simulink model "rlMultiAgentPFC"  (R2022a)
settings: Solver=VariableStepAuto  StartTime=0.0  StopTime=Tf  FixedStep=1e-3  RelTol=1e-3
values from neighbouring files (symbols this model uses):
  Ts = 100    [MultiAgent_initiateSAC.m]    (also in control_velocity.m; initiate.m; initiateHybrid.m = 50; initiateSAC.m)
undefined symbols (not defined in the file or in its folder): amax_ego, amin_ego, Cf, Cr, D_default, DiscIntNeverNeededParam, e1_initial, e2_initial, Iz, lf, lr, m, rho, t_gap, tau, umax_ego, umin_ego, v0_ego, v0_lead, v_set, x0_ego, x0_lead
libraries: simulink x5, rllib x2
settings Model: Creator=The MathWorks, Inc.  LastModifiedBy=The MathWorks, Inc.
settings SolverCC: AlgebraicLoopSolver=TrustRegion
settings DataIOCC: SaveOutput=off  SignalLogging=off  DSMLogging=off  SaveTime=off  ReturnWorkspaceOutputs=off
settings DebuggingCC: ParameterPrecisionLossMsg=none  UnconnectedInputMsg=warning  UnconnectedOutputMsg=warning  UnconnectedLineMsg=warning  SFMachineParentedDataDiag=warning  ArithmeticOperatorsInVariantConditions=warning
settings SFSimCC: SimUseLocalCustomCode=off
settings RTWCC: RTWUseLocalCustomCode=off  DLArmComputeVersion=19.05

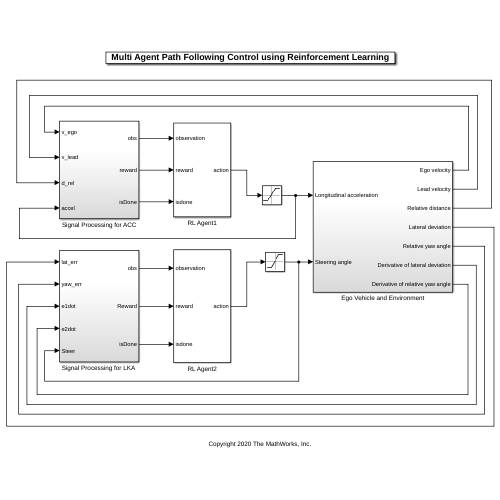
[thumbnail: Simulink's stored preview of the top-level diagram]
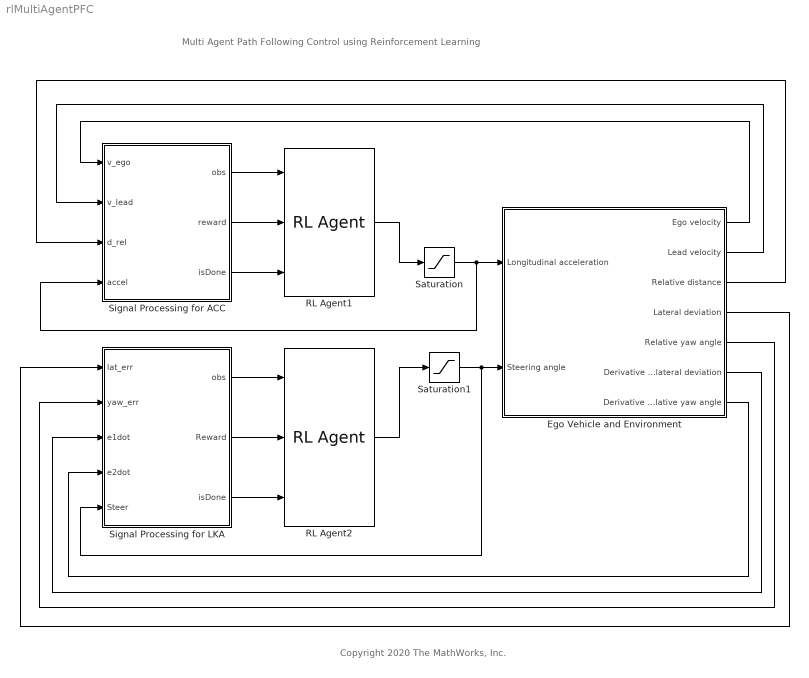
== system rlMultiAgentPFC ==
  note: Copyright 2020 The MathWorks, Inc.
  note: Multi Agent Path Following Control using Reinforcement Learning
  Ego Vehicle and Environment : Subsystem
  RL Agent1 : rllib/RL Agent  Agent=agent1  ExternalActionAsInput=off  ProvideLastAction=off  ProvideCumRwd=off  TreatAsDirectFeedthrough=on  UseStrictObservationDataTypes=off
  RL Agent2 : rllib/RL Agent  Agent=agent2  ExternalActionAsInput=off  ProvideLastAction=off  ProvideCumRwd=off  TreatAsDirectFeedthrough=on  UseStrictObservationDataTypes=off
  Saturation : Saturate  UpperLimit=amax_ego  LowerLimit=amin_ego
  Saturation1 : Saturate  UpperLimit=umax_ego  LowerLimit=umin_ego
  Signal Processing for ACC : Subsystem
  "Signal Processing for LKA " : Subsystem
  wires:
  Saturation/1 -> Signal Processing for ACC/4(accel), Ego Vehicle and Environment/1(Longitudinal acceleration)
  Saturation1/1 -> "Signal Processing for LKA "/5(Steer), Ego Vehicle and Environment/2(Steering angle)
  RL Agent1/1 -> Saturation/1
  RL Agent2/1 -> Saturation1/1
  Signal Processing for ACC/1(obs) -> RL Agent1/1
  Signal Processing for ACC/2(reward) -> RL Agent1/2
  Signal Processing for ACC/3(isDone) -> RL Agent1/3
  "Signal Processing for LKA "/1(obs) -> RL Agent2/1
  "Signal Processing for LKA "/2(Reward) -> RL Agent2/2
  "Signal Processing for LKA "/3(isDone) -> RL Agent2/3
  Ego Vehicle and Environment/3(Relative distance) -> Signal Processing for ACC/3(d_rel)
  Ego Vehicle and Environment/2(Lead velocity) -> Signal Processing for ACC/2(v_lead)
  Ego Vehicle and Environment/1(Ego velocity) -> Signal Processing for ACC/1(v_ego)
  Ego Vehicle and Environment/7(Derivative of relative yaw angle) -> "Signal Processing for LKA "/4(e2dot)
  Ego Vehicle and Environment/6(Derivative of lateral deviation) -> "Signal Processing for LKA "/3("e1dot ")
  Ego Vehicle and Environment/5(Relative yaw angle) -> "Signal Processing for LKA "/2(yaw_err)
  Ego Vehicle and Environment/4(Lateral deviation) -> "Signal Processing for LKA "/1(lat_err)

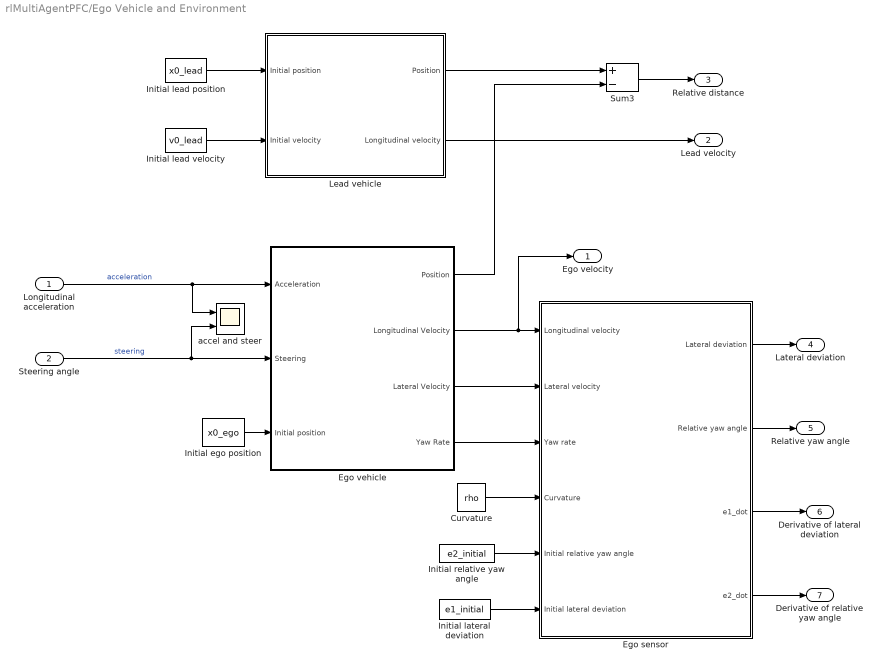
== system rlMultiAgentPFC/Ego Vehicle and Environment ==
  Longitudinal acceleration : Inport
  Steering angle : Inport  Port=2
  Curvature : Constant  Value=rho
  Ego sensor : Subsystem
  Ego vehicle : Subsystem
  Initial ego position : Constant  Value=x0_ego
  Initial lateral deviation : Constant  Value=e1_initial
  Initial lead position : Constant  Value=x0_lead
  Initial lead velocity : Constant  Value=v0_lead
  Initial relative yaw angle : Constant  Value=e2_initial
  Lead vehicle : Subsystem
  Sum3 : Sum  Inputs=+-
  accel and steer : Scope  NumInputPorts=2
  Ego velocity : Outport  VectorParamsAs1DForOutWhenUnconnected=off
  Lead velocity : Outport  Port=2  VectorParamsAs1DForOutWhenUnconnected=off
  Relative distance : Outport  Port=3  VectorParamsAs1DForOutWhenUnconnected=off
  Lateral deviation : Outport  Port=4  VectorParamsAs1DForOutWhenUnconnected=off
  Relative yaw angle : Outport  Port=5  VectorParamsAs1DForOutWhenUnconnected=off
  Derivative of lateral deviation : Outport  Port=6  VectorParamsAs1DForOutWhenUnconnected=off
  Derivative of relative yaw angle : Outport  Port=7  VectorParamsAs1DForOutWhenUnconnected=off
  wires:
  Ego vehicle/3(Lateral Velocity) -> Ego sensor/2(Lateral velocity)
  Ego vehicle/4(Yaw Rate) -> Ego sensor/3(Yaw rate)
  Longitudinal acceleration/1 -> accel and steer/1, Ego vehicle/1(Acceleration)  "acceleration"
  Ego sensor/1(Lateral deviation) -> Lateral deviation/1
  Ego vehicle/2(Longitudinal Velocity) -> Ego velocity/1, Ego sensor/1(Longitudinal velocity)
  Steering angle/1 -> accel and steer/2, Ego vehicle/2(Steering)  "steering"
  Ego sensor/2(Relative yaw angle) -> Relative yaw angle/1
  Initial lateral deviation/1 -> Ego sensor/6(Initial lateral deviation)
  Initial ego position/1 -> Ego vehicle/3(Initial position)
  Curvature/1 -> Ego sensor/4(Curvature)
  Initial relative yaw angle/1 -> Ego sensor/5(Initial relative yaw angle)
  Initial lead velocity/1 -> Lead vehicle/2(Initial velocity)
  Initial lead position/1 -> Lead vehicle/1(Initial position)
  Lead vehicle/1(Position) -> Sum3/1
  Ego vehicle/1(Position) -> Sum3/2
  Sum3/1 -> Relative distance/1
  Lead vehicle/2(Longitudinal velocity) -> Lead velocity/1
  Ego sensor/3(e1_dot) -> Derivative of lateral deviation/1
  Ego sensor/4(e2_dot) -> Derivative of relative yaw angle/1

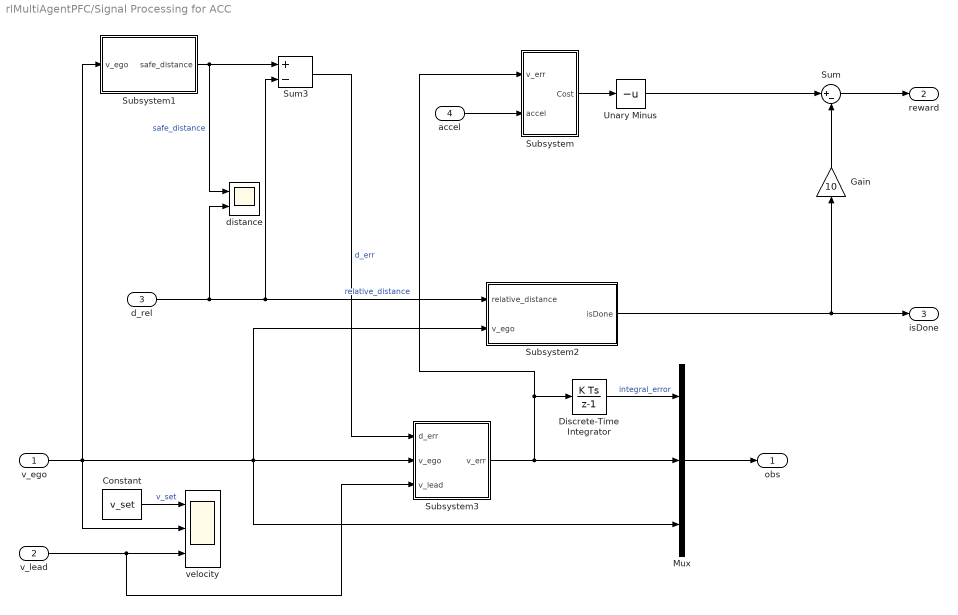
== system rlMultiAgentPFC/Signal Processing for ACC ==
  v_ego : Inport
  v_lead : Inport  Port=2
  d_rel : Inport  Port=3
  accel : Inport  Port=4
  Constant : Constant  Value=v_set
  Discrete-Time Integrator : DiscreteIntegrator  SampleTime=-1  ICPrevOutput=DiscIntNeverNeededParam  ICPrevScaledInput=DiscIntNeverNeededParam
  Gain : Gain  Gain=10
  Mux : Mux  Inputs=3
  Subsystem : Subsystem
  Subsystem1 : Subsystem
  Subsystem2 : Subsystem
  Subsystem3 : Subsystem
  Sum : Sum  Inputs=|+-
  Sum3 : Sum  Inputs=+-
  Unary Minus : UnaryMinus
  distance : Scope  NumInputPorts=2
  velocity : Scope  NumInputPorts=3
  obs : Outport  VectorParamsAs1DForOutWhenUnconnected=off
  reward : Outport  Port=2  VectorParamsAs1DForOutWhenUnconnected=off
  isDone : Outport  Port=3  VectorParamsAs1DForOutWhenUnconnected=off
  wires:
  Constant/1 -> velocity/1  "v_set"
  v_lead/1 -> velocity/3, Subsystem3/3(v_lead)
  Discrete-Time Integrator/1 -> Mux/1  "integral_error"
  Mux/1 -> obs/1
  v_ego/1 -> velocity/2, Subsystem3/2(v_ego), Mux/3, Subsystem2/2(v_ego), Subsystem1/1(v_ego)
  d_rel/1 -> distance/2, Sum3/2, Subsystem2/1(relative_distance)  "relative_distance"
  Subsystem/1(Cost) -> Unary Minus/1
  Sum3/1 -> Subsystem3/1(d_err)  "d_err"
  Subsystem1/1(safe_distance) -> distance/1, Sum3/1  "safe_distance"
  accel/1 -> Subsystem/2(accel)
  Subsystem3/1(v_err) -> Subsystem/1(v_err), Discrete-Time Integrator/1, Mux/2
  Subsystem2/1(isDone) -> isDone/1, Gain/1
  Unary Minus/1 -> Sum/1
  Gain/1 -> Sum/2
  Sum/1 -> reward/1

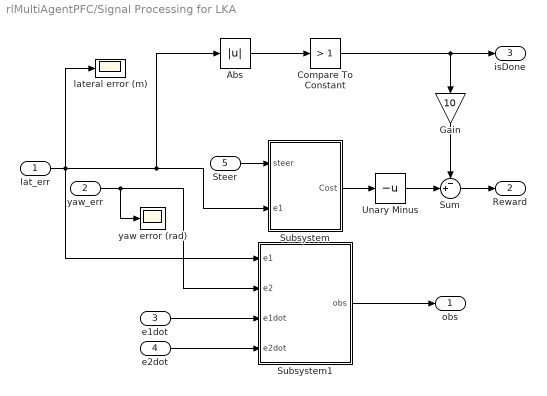
== system rlMultiAgentPFC/Signal Processing for LKA  ==
  lat_err : Inport
  yaw_err : Inport  Port=2
  "e1dot " : Inport  Port=3
  e2dot : Inport  Port=4
  Steer : Inport  Port=5
  Abs : Abs  SaturateOnIntegerOverflow=off
  Compare To Constant : simulink/Logic and Bit Operations/Compare To Constant  relop=>  const=1  OutDataTypeStr=boolean
  Gain : Gain  Gain=10
  Subsystem : Subsystem
  Subsystem1 : Subsystem
  Sum : Sum  Inputs=-+|
  Unary Minus : UnaryMinus
  lateral error (m) : Scope
  yaw error (rad) : Scope
  obs : Outport  VectorParamsAs1DForOutWhenUnconnected=off
  Reward : Outport  Port=2  VectorParamsAs1DForOutWhenUnconnected=off
  isDone : Outport  Port=3  VectorParamsAs1DForOutWhenUnconnected=off
  wires:
  Subsystem/1(Cost) -> Unary Minus/1
  lat_err/1 -> Subsystem1/1(e1), Subsystem/2(e1), Abs/1, lateral error (m)/1
  yaw_err/1 -> yaw error (rad)/1, Subsystem1/2(e2)
  Abs/1 -> Compare To Constant/1
  Subsystem1/1(obs) -> obs/1
  "e1dot "/1 -> Subsystem1/3(e1dot)
  e2dot/1 -> Subsystem1/4(e2dot)
  Steer/1 -> Subsystem/1(steer)
  Compare To Constant/1 -> Gain/1, isDone/1
  Gain/1 -> Sum/1
  Sum/1 -> Reward/1
  Unary Minus/1 -> Sum/2

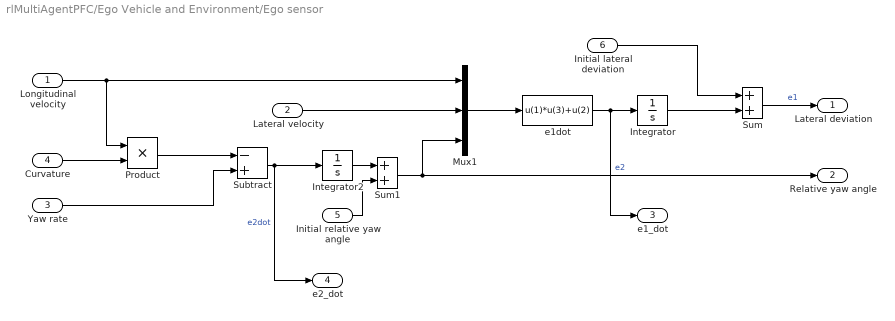
== system rlMultiAgentPFC/Ego Vehicle and Environment/Ego sensor ==
  Longitudinal velocity : Inport
  Lateral velocity : Inport  Port=2
  Yaw rate : Inport  Port=3
  Curvature : Inport  Port=4
  Initial relative yaw angle : Inport  Port=5
  Initial lateral deviation : Inport  Port=6
  Integrator : Integrator
  Integrator2 : Integrator
  Mux1 : Mux  Inputs=[1 1 1]
  Product : Product
  Subtract : Sum  Inputs=-+
  Sum : Sum
  Sum1 : Sum
  e1dot : Fcn  Expr=u(1)*u(3)+u(2)
  Lateral deviation : Outport  VectorParamsAs1DForOutWhenUnconnected=off
  Relative yaw angle : Outport  Port=2  VectorParamsAs1DForOutWhenUnconnected=off
  e1_dot : Outport  Port=3  VectorParamsAs1DForOutWhenUnconnected=off
  e2_dot : Outport  Port=4  VectorParamsAs1DForOutWhenUnconnected=off
  wires:
  Curvature/1 -> Product/2
  Sum1/1 -> Mux1/3, Relative yaw angle/1  "e2"
  Mux1/1 -> e1dot/1
  Initial lateral deviation/1 -> Sum/1
  e1dot/1 -> e1_dot/1, Integrator/1
  Integrator/1 -> Sum/2
  Longitudinal velocity/1 -> Product/1, Mux1/1
  Lateral velocity/1 -> Mux1/2
  Sum/1 -> Lateral deviation/1  "e1"
  Integrator2/1 -> Sum1/1
  Initial relative yaw angle/1 -> Sum1/2
  Product/1 -> Subtract/1
  Yaw rate/1 -> Subtract/2
  Subtract/1 -> e2_dot/1, Integrator2/1  "e2dot"

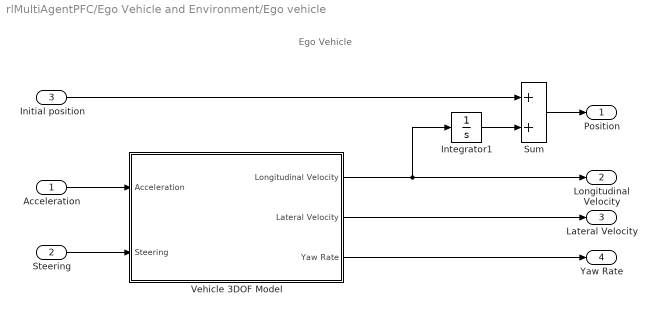
== system rlMultiAgentPFC/Ego Vehicle and Environment/Ego vehicle ==
  note: Ego Vehicle
  Acceleration : Inport
  Steering : Inport  Port=2
  Initial position : Inport  Port=3
  Integrator1 : Integrator
  Sum : Sum
  Vehicle 3DOF Model : Subsystem
  Position : Outport  VectorParamsAs1DForOutWhenUnconnected=off
  Longitudinal Velocity : Outport  Port=2  VectorParamsAs1DForOutWhenUnconnected=off
  Lateral Velocity : Outport  Port=3  VectorParamsAs1DForOutWhenUnconnected=off
  Yaw Rate : Outport  Port=4  VectorParamsAs1DForOutWhenUnconnected=off
  wires:
  Integrator1/1 -> Sum/2
  Initial position/1 -> Sum/1
  Sum/1 -> Position/1
  Acceleration/1 -> Vehicle 3DOF Model/1(Acceleration)
  Steering/1 -> Vehicle 3DOF Model/2(Steering)
  Vehicle 3DOF Model/2(Lateral Velocity) -> Lateral Velocity/1
  Vehicle 3DOF Model/3(Yaw Rate) -> Yaw Rate/1
  Vehicle 3DOF Model/1(Longitudinal Velocity) -> Longitudinal Velocity/1, Integrator1/1

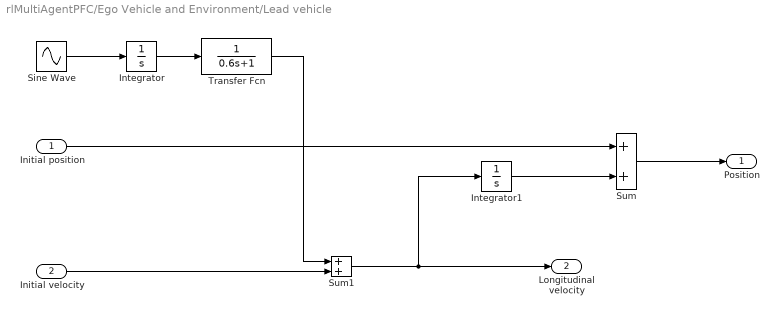
== system rlMultiAgentPFC/Ego Vehicle and Environment/Lead vehicle ==
  Initial position : Inport
  Initial velocity : Inport  Port=2
  Integrator : Integrator
  Integrator1 : Integrator
  Sine Wave : Sin  Amplitude=0.6  Frequency=0.2  SampleTime=Ts
  Sum : Sum
  Sum1 : Sum
  Transfer Fcn : TransferFcn  Denominator=[0.6 1]
  Position : Outport  VectorParamsAs1DForOutWhenUnconnected=off
  Longitudinal velocity : Outport  Port=2  VectorParamsAs1DForOutWhenUnconnected=off
  wires:
  Transfer Fcn/1 -> Sum1/1
  Initial velocity/1 -> Sum1/2
  Sum/1 -> Position/1
  Integrator/1 -> Transfer Fcn/1
  Sum1/1 -> Integrator1/1, Longitudinal velocity/1
  Sine Wave/1 -> Integrator/1
  Initial position/1 -> Sum/1
  Integrator1/1 -> Sum/2

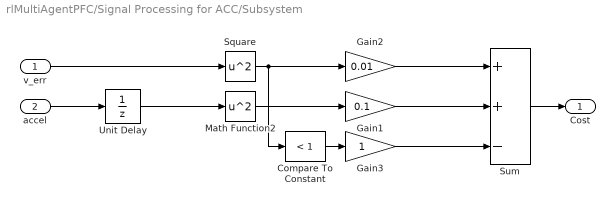
== system rlMultiAgentPFC/Signal Processing for ACC/Subsystem ==
  v_err : Inport
  accel : Inport  Port=2
  Compare To Constant : simulink/Logic and Bit Operations/Compare To Constant  relop=<  const=1  OutDataTypeStr=boolean
  Gain1 : Gain  Gain=0.1
  Gain2 : Gain  Gain=0.01
  Gain3 : Gain
  Math Function2 : Math  Operator=square  SignedPower=on
  Square : Math  Operator=square  SignedPower=on
  Sum : Sum  Inputs=++-
  Unit Delay : UnitDelay  SampleTime=-1  HasFrameUpgradeWarning=on
  Cost : Outport  VectorParamsAs1DForOutWhenUnconnected=off
  wires:
  v_err/1 -> Square/1
  Math Function2/1 -> Gain1/1
  accel/1 -> Unit Delay/1
  Sum/1 -> Cost/1
  Square/1 -> Compare To Constant/1, Gain2/1
  Unit Delay/1 -> Math Function2/1
  Gain2/1 -> Sum/1
  Gain1/1 -> Sum/2
  Compare To Constant/1 -> Gain3/1
  Gain3/1 -> Sum/3

== system rlMultiAgentPFC/Signal Processing for ACC/Subsystem1 ==
  v_ego : Inport
  Default Spacing : Constant  Value=D_default  SampleTime=Ts
  Product : Product
  Sum2 : Sum
  Time Gap : Constant  Value=t_gap  SampleTime=Ts
  safe_distance : Outport  VectorParamsAs1DForOutWhenUnconnected=off
  wires:
  Sum2/1 -> safe_distance/1
  Product/1 -> Sum2/2
  Time Gap/1 -> Product/2
  Default Spacing/1 -> Sum2/1
  v_ego/1 -> Product/1

== system rlMultiAgentPFC/Signal Processing for ACC/Subsystem2 ==
  relative_distance : Inport
  v_ego : Inport  Port=2
  Logical Operator : Logic  Operator=OR  AllPortsSameDT=off  OutDataTypeStr=boolean
  Relative Distance : simulink/Logic and Bit Operations/Compare To Constant  relop=<  const=0  OutDataTypeStr=boolean
  Velocity : simulink/Logic and Bit Operations/Compare To Constant  relop=<  const=0.5  OutDataTypeStr=boolean
  isDone : Outport  VectorParamsAs1DForOutWhenUnconnected=off
  wires:
  Velocity/1 -> Logical Operator/2
  Relative Distance/1 -> Logical Operator/1
  relative_distance/1 -> Relative Distance/1
  Logical Operator/1 -> isDone/1
  v_ego/1 -> Velocity/1

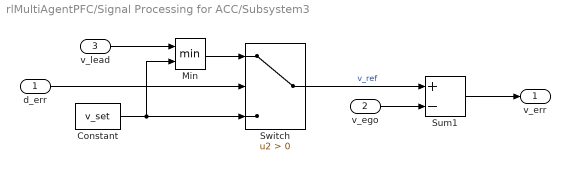
== system rlMultiAgentPFC/Signal Processing for ACC/Subsystem3 ==
  d_err : Inport
  v_ego : Inport  Port=2
  v_lead : Inport  Port=3
  Constant : Constant  Value=v_set
  Min : MinMax  Inputs=2
  Sum1 : Sum  Inputs=+-
  Switch : Switch  Criteria=u2 > Threshold  SaturateOnIntegerOverflow=off  InputSameDT=off
  v_err : Outport  VectorParamsAs1DForOutWhenUnconnected=off
  wires:
  Sum1/1 -> v_err/1
  v_ego/1 -> Sum1/2
  Switch/1 -> Sum1/1  "v_ref"
  d_err/1 -> Switch/2
  Constant/1 -> Min/2, Switch/3
  Min/1 -> Switch/1
  v_lead/1 -> Min/1

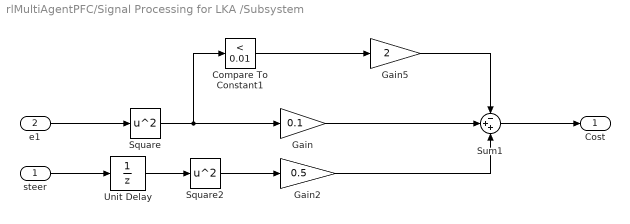
== system rlMultiAgentPFC/Signal Processing for LKA /Subsystem ==
  steer : Inport
  e1 : Inport  Port=2
  Compare To Constant1 : simulink/Logic and Bit Operations/Compare To Constant  relop=<  const=0.01  OutDataTypeStr=boolean
  Gain : Gain  Gain=0.1
  Gain2 : Gain  Gain=0.5
  Gain5 : Gain  Gain=2
  Square : Math  Operator=square  SignedPower=on
  Square2 : Math  Operator=square  SignedPower=on
  Sum1 : Sum  Inputs=-++
  Unit Delay : UnitDelay  SampleTime=-1  HasFrameUpgradeWarning=on
  Cost : Outport  VectorParamsAs1DForOutWhenUnconnected=off
  wires:
  e1/1 -> Square/1
  Sum1/1 -> Cost/1
  Gain/1 -> Sum1/2
  steer/1 -> Unit Delay/1
  Square2/1 -> Gain2/1
  Gain2/1 -> Sum1/3
  Unit Delay/1 -> Square2/1
  Compare To Constant1/1 -> Gain5/1
  Square/1 -> Compare To Constant1/1, Gain/1
  Gain5/1 -> Sum1/1

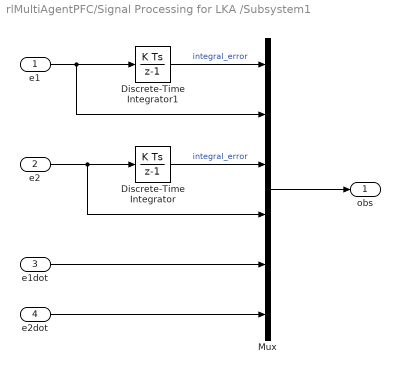
== system rlMultiAgentPFC/Signal Processing for LKA /Subsystem1 ==
  e1 : Inport
  e2 : Inport  Port=2
  e1dot : Inport  Port=3
  e2dot : Inport  Port=4
  Discrete-Time Integrator : DiscreteIntegrator  SampleTime=-1  ICPrevOutput=DiscIntNeverNeededParam  ICPrevScaledInput=DiscIntNeverNeededParam
  Discrete-Time Integrator1 : DiscreteIntegrator  SampleTime=-1  ICPrevOutput=DiscIntNeverNeededParam  ICPrevScaledInput=DiscIntNeverNeededParam
  Mux : Mux  Inputs=6
  obs : Outport  VectorParamsAs1DForOutWhenUnconnected=off
  wires:
  e1/1 -> Mux/2, Discrete-Time Integrator1/1
  Mux/1 -> obs/1
  Discrete-Time Integrator1/1 -> Mux/1  "integral_error"
  e2/1 -> Mux/4, Discrete-Time Integrator/1
  Discrete-Time Integrator/1 -> Mux/3  "integral_error"
  e1dot/1 -> Mux/5
  e2dot/1 -> Mux/6

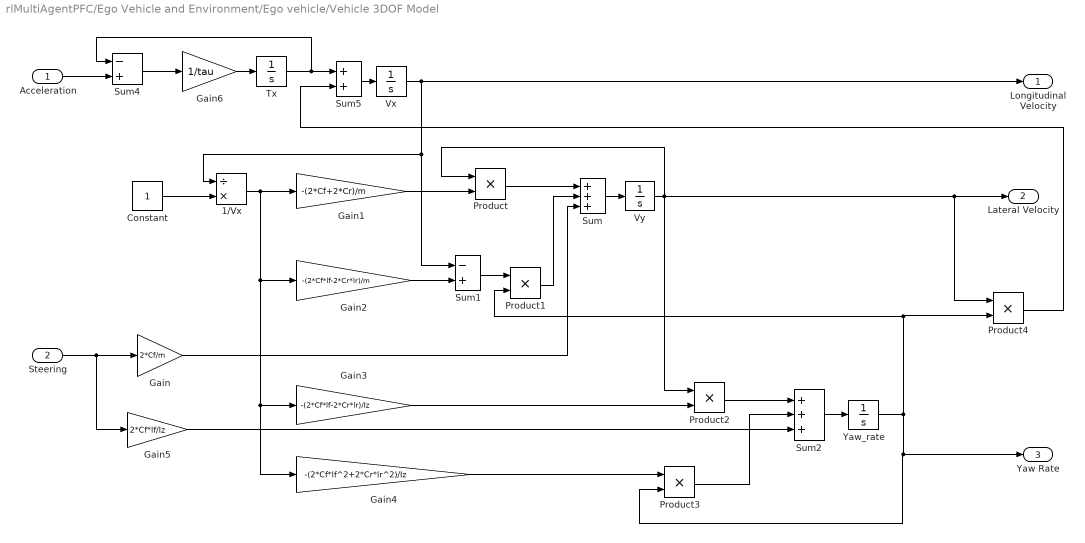
== system rlMultiAgentPFC/Ego Vehicle and Environment/Ego vehicle/Vehicle 3DOF Model ==
  Acceleration : Inport
  Steering : Inport  Port=2
  1/Vx : Product  Inputs=/*
  Constant : Constant
  Gain : Gain  Gain=2*Cf/m
  Gain1 : Gain  Gain=-(2*Cf+2*Cr)/m
  Gain2 : Gain  Gain=-(2*Cf*lf-2*Cr*lr)/m
  Gain3 : Gain  Gain=-(2*Cf*lf-2*Cr*lr)/Iz
  Gain4 : Gain  Gain=-(2*Cf*lf^2+2*Cr*lr^2)/Iz
  Gain5 : Gain  Gain=2*Cf*lf/Iz
  Gain6 : Gain  Gain=1/tau
  Product{,1..4} (5 alike) : Product
  Sum : Sum  Inputs=+++
  Sum1 : Sum  Inputs=-+
  Sum2 : Sum  Inputs=+++
  Sum4 : Sum  Inputs=-+
  Sum5 : Sum
  Tx : Integrator
  Vx : Integrator  InitialCondition=v0_ego
  Vy : Integrator
  "Yaw_rate " : Integrator
  Longitudinal Velocity : Outport  VectorParamsAs1DForOutWhenUnconnected=off
  Lateral Velocity : Outport  Port=2  VectorParamsAs1DForOutWhenUnconnected=off
  Yaw Rate : Outport  Port=3  VectorParamsAs1DForOutWhenUnconnected=off
  wires:
  Vy/1 -> Product/1, Lateral Velocity/1, Product4/1, Product2/1
  Gain2/1 -> Sum1/2
  Product/1 -> Sum/1
  Tx/1 -> Sum5/1, Sum4/1
  Sum/1 -> Vy/1
  "Yaw_rate "/1 -> Yaw Rate/1, Product3/2, Product4/2, Product1/2
  1/Vx/1 -> Gain4/1, Gain3/1, Gain2/1, Gain1/1
  Vx/1 -> 1/Vx/1, Sum1/1, Longitudinal Velocity/1
  Product3/1 -> Sum2/2
  Steering/1 -> Gain/1, Gain5/1
  Acceleration/1 -> Sum4/2
  Sum1/1 -> Product1/1
  Gain/1 -> Sum/3
  Gain1/1 -> Product/2
  Gain6/1 -> Tx/1
  Product2/1 -> Sum2/1
  Sum5/1 -> Vx/1
  Constant/1 -> 1/Vx/2
  Product1/1 -> Sum/2
  Sum4/1 -> Gain6/1
  Gain4/1 -> Product3/1
  Product4/1 -> Sum5/2
  Gain3/1 -> Product2/2
  Gain5/1 -> Sum2/3
  Sum2/1 -> "Yaw_rate "/1
